simulink model "velocity_control"  (R2015a)
settings: Solver=ode45  StartTime=0.0  StopTime=10.0  RelTol=1e-3
values from neighbouring files (symbols this model uses):
  Kvp = 4    [pi_and_ip.m]
  m = 1    [pi_and_ip.m]    (also in velocity_control_matlab.m = 1;'})
settings Model: Creator=shohei  LastModifiedBy=shohei

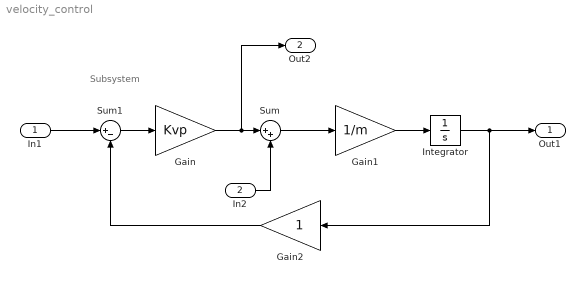
== system velocity_control ==
  note: Subsystem
  In1 : Inport
  In2 : Inport  Port=2
  Gain : Gain  Gain=Kvp
  Gain1 : Gain  Gain=1/m
  Gain2 : Gain
  Integrator : Integrator
  Sum : Sum  Inputs=|++
  Sum1 : Sum  Inputs=|+-
  Out1 : Outport
  Out2 : Outport  Port=2
  wires:
  Integrator/1 -> Out1/1, Gain2/1
  Gain2/1 -> Sum1/2
  Gain/1 -> Out2/1, Sum/1
  In1/1 -> Sum1/1
  Sum/1 -> Gain1/1
  Gain1/1 -> Integrator/1
  In2/1 -> Sum/2
  Sum1/1 -> Gain/1
